simulink model "parte2"  (R2017b)
settings: Solver=VariableStepAuto  StartTime=0.0  StopTime=10.0  RelTol=1e-3
libraries: simulink x2
settings Model: Creator=zeroz  LastModifiedBy=zeroz

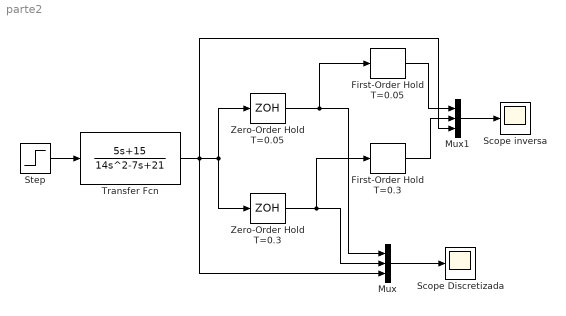
== system parte2 ==
  First-Order Hold T=0.05 : simulink/Discrete/First-Order Hold  DisableCoverage=on  Ts=0.05
      settings: SourceProductName=Simulink  SourceProductBaseCode=SL
  "First-Order Hold T=0.3 " : simulink/Discrete/First-Order Hold  DisableCoverage=on  Ts=0.3
      settings: SourceProductName=Simulink  SourceProductBaseCode=SL
  Mux : Mux  Inputs=3
  Mux1 : Mux  Inputs=3
  Scope Discretizada : Scope
  Scope inversa : Scope
  Step : Step  SampleTime=0
  Transfer Fcn : TransferFcn  Numerator=[5 15]  Denominator=[14 -7 21]
  Zero-Order Hold T=0.05 : ZeroOrderHold  SampleTime=0.05
  Zero-Order Hold T=0.3 : ZeroOrderHold  SampleTime=0.3
  wires:
  Step/1 -> Transfer Fcn/1
  Transfer Fcn/1 -> Mux1/3, Mux/3, Zero-Order Hold T=0.3/1, Zero-Order Hold T=0.05/1
  Zero-Order Hold T=0.3/1 -> "First-Order Hold T=0.3 "/1, Mux/2
  Zero-Order Hold T=0.05/1 -> First-Order Hold T=0.05/1, Mux/1
  First-Order Hold T=0.05/1 -> Mux1/1
  "First-Order Hold T=0.3 "/1 -> Mux1/2
  Mux/1 -> Scope Discretizada/1
  Mux1/1 -> Scope inversa/1
